simulink model "mass_damper_system"  (R2021b)
settings: Solver=VariableStepAuto  StartTime=0.0  StopTime=30  RelTol=1e-3
values from neighbouring files (symbols this model uses):
  C = (s + 0.2) / (s + 0.11)    [Lag_compensator.m]    (also in PD_controller.m = Kp + Kd*s; P_controller.m = 10; lag_lead_compensator.m = ((s + 0.1)/(s + 0.01)) * ((s + 10)/(s + 100)))
  K = 0.01    [simscapeParameters.m]    (also in simscapeVisualization.m)
undefined symbols (not defined in the file or in its folder): F, M
libraries: aerolibanimutils x1
settings Model: Creator=Joshua  LastModifiedBy=Joshua

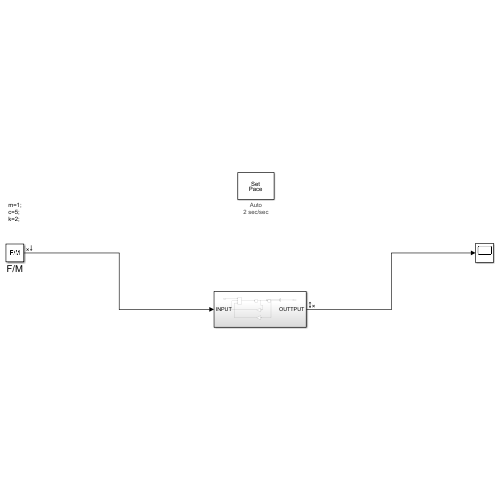
[thumbnail: Simulink's stored preview of the top-level diagram]
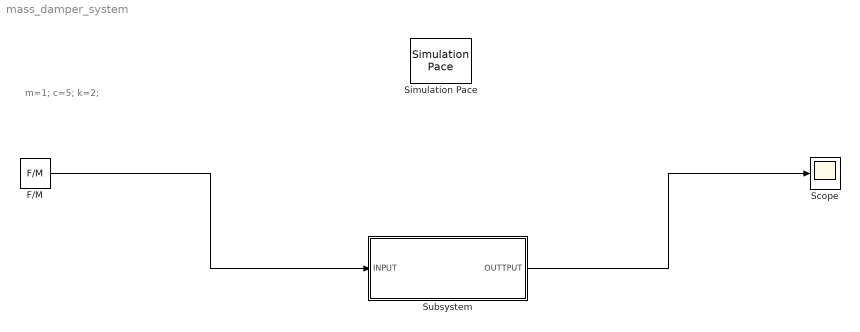
== system mass_damper_system ==
  note: m=1;
      | c=5;
      | k=2;
  F/M : Constant  Value=F/M
  Scope : Scope
  Simulation Pace : aerolibanimutils/Simulation Pace  SimulationPace=2  SleepMode=Auto  OutputPaceError=off  SampleTime=1/30
  Subsystem : Subsystem
  wires:
  F/M/1 -> Subsystem/1(INPUT)
  Subsystem/1(OUTTPUT) -> Scope/1

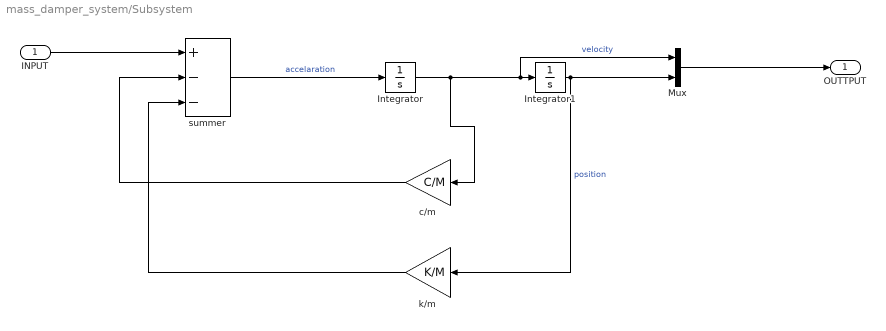
== system mass_damper_system/Subsystem ==
  INPUT : Inport
  Integrator : Integrator
  Integrator1 : Integrator
  Mux : Mux  Inputs=2
  c/m : Gain  Gain=C/M
  k/m : Gain  Gain=K/M
  summer : Sum  Inputs=+--
  OUTTPUT : Outport
  wires:
  summer/1 -> Integrator/1  "accelaration"
  Integrator/1 -> c/m/1, Mux/1, Integrator1/1  "velocity"
  c/m/1 -> summer/2
  Integrator1/1 -> k/m/1, Mux/2  "position"
  INPUT/1 -> summer/1
  k/m/1 -> summer/3
  Mux/1 -> OUTTPUT/1
